simulink library "half_bridge_LLC_modulator"  (R2025b)
settings: Solver=VariableStepAuto  StartTime=0.0  StopTime=10.0  RelTol=1e-3
undefined symbols (not defined in the file): tc
settings Model: Creator=dbagn  LastModifiedBy=dbagn

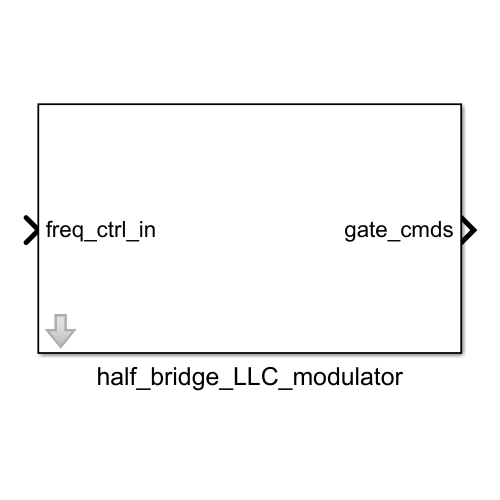
[thumbnail: Simulink's stored preview of the top-level diagram]
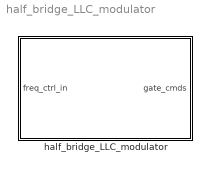
== system half_bridge_LLC_modulator ==
  half_bridge_LLC_modulator : Subsystem  mask{fPWM_max=100e3, fres=116e3}
      mask prompts: fPWM_max "fPWM_max [Hz]"; fres "Resonance frequency [Hz]"

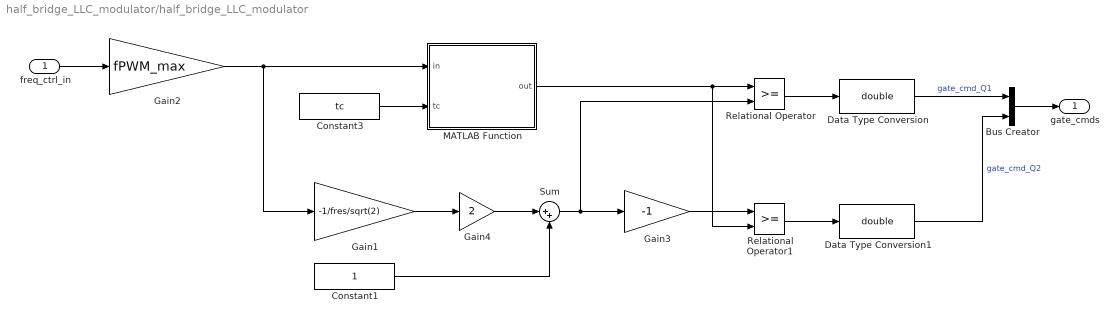
== system half_bridge_LLC_modulator/half_bridge_LLC_modulator ==
  freq_ctrl_in : Inport
  Bus Creator : BusCreator  Inputs=2
  Constant1 : Constant
  Constant3 : Constant  Value=tc
  Data Type Conversion : DataTypeConversion  OutDataTypeStr=double  SaturateOnIntegerOverflow=off  RndMeth=Floor
  Data Type Conversion1 : DataTypeConversion  OutDataTypeStr=double  SaturateOnIntegerOverflow=off  RndMeth=Floor
  Gain1 : Gain  Gain=-1/fres/sqrt(2)  OutDataTypeStr=double
  Gain2 : Gain  Gain=fPWM_max  OutDataTypeStr=double
  Gain3 : Gain  Gain=-1  OutDataTypeStr=double
  Gain4 : Gain  Gain=2  OutDataTypeStr=double
  MATLAB Function : MATLAB Function  TreatAsAtomicUnit=on  SystemSampleTime=tc
  Relational Operator : RelationalOperator
  Relational Operator1 : RelationalOperator
  Sum : Sum  Inputs=|++
  gate_cmds : Outport
  wires:
  freq_ctrl_in/1 -> Gain2/1
  MATLAB Function/1(out) -> Relational Operator1/2, Relational Operator/1
  Constant3/1 -> MATLAB Function/2(tc)
  Relational Operator/1 -> Data Type Conversion/1
  Data Type Conversion/1 -> Bus Creator/1  "gate_cmd_Q1"
  Data Type Conversion1/1 -> Bus Creator/2  "gate_cmd_Q2"
  Gain2/1 -> Gain1/1, MATLAB Function/1(in)
  Gain1/1 -> Gain4/1
  Sum/1 -> Gain3/1, Relational Operator/2
  Constant1/1 -> Sum/2
  Gain3/1 -> Relational Operator1/1
  Relational Operator1/1 -> Data Type Conversion1/1
  Gain4/1 -> Sum/1
  Bus Creator/1 -> gate_cmds/1

== matlab function half_bridge_LLC_modulator/MATLAB Function ==
  data: in input; out output; tc input
function out = triangle(in,tc)

persistent y k

if isempty(y)
    y = 0;
    k = 1;
end

if y > 1
    k = -1;
    y = y + 4*k * in * tc;
elseif y < -1
    k = 1;
    y = y + 4*k * in * tc;
else
    y = y + 4*k * in * tc;
end
out = y;
